simulink model "problem_7"  (R2020b)
settings: Solver=VariableStepAuto  StartTime=0.0  StopTime=10.0  RelTol=1e-3
values from neighbouring files (symbols this model uses):
  b11 = 1    [vars.m]
  b12 = 2    [vars.m]
  b13 = 1    [vars.m]
  b21 = 1    [vars.m]
  b22 = 1    [vars.m]
settings Model: Creator=hp  LastModifiedBy=hp

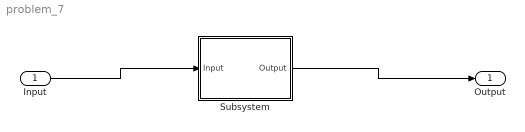
== system problem_7 ==
  Input : Inport
  Subsystem : Subsystem
  Output : Outport
  wires:
  Input/1 -> Subsystem/1(Input)
  Subsystem/1(Output) -> Output/1

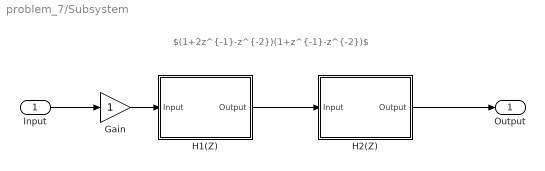
== system problem_7/Subsystem ==
  note: $(1+2z^{-1}-z^{-2})(1+z^{-1}-z^{-2})$
  Input : Inport
  Gain : Gain
  H1(Z) : Subsystem
  H2(Z) : Subsystem
  Output : Outport
  wires:
  H1(Z)/1(Output) -> H2(Z)/1(Input)
  H2(Z)/1(Output) -> Output/1
  Input/1 -> Gain/1
  Gain/1 -> H1(Z)/1(Input)

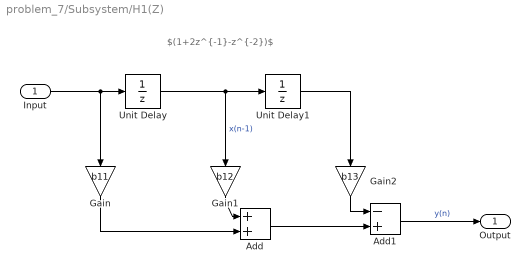
== system problem_7/Subsystem/H1(Z) ==
  note: $(1+2z^{-1}-z^{-2})$
  Input : Inport
  Add : Sum
  Add1 : Sum  Inputs=-+
  Gain : Gain  Gain=b11
  Gain1 : Gain  Gain=b12
  Gain2 : Gain  Gain=b13
  Unit Delay : UnitDelay  SampleTime=-1  HasFrameUpgradeWarning=on
  Unit Delay1 : UnitDelay  SampleTime=-1  HasFrameUpgradeWarning=on
  Output : Outport
  wires:
  Unit Delay1/1 -> Gain2/1
  Gain1/1 -> Add/1
  Add/1 -> Add1/2
  Gain/1 -> Add/2
  Unit Delay/1 -> Gain1/1, Unit Delay1/1  "x(n-1)"
  Input/1 -> Gain/1, Unit Delay/1
  Gain2/1 -> Add1/1
  Add1/1 -> Output/1  "y(n)"

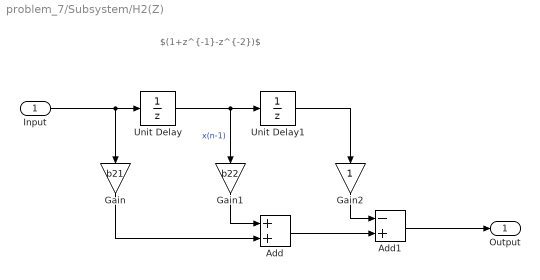
== system problem_7/Subsystem/H2(Z) ==
  note: $(1+z^{-1}-z^{-2})$
  Input : Inport
  Add : Sum
  Add1 : Sum  Inputs=-+
  Gain : Gain  Gain=b21
  Gain1 : Gain  Gain=b22
  Gain2 : Gain
  Unit Delay : UnitDelay  SampleTime=-1  HasFrameUpgradeWarning=on
  Unit Delay1 : UnitDelay  SampleTime=-1  HasFrameUpgradeWarning=on
  Output : Outport
  wires:
  Unit Delay/1 -> Gain1/1, Unit Delay1/1  "x(n-1)"
  Input/1 -> Gain/1, Unit Delay/1
  Add1/1 -> Output/1
  Gain/1 -> Add/2
  Unit Delay1/1 -> Gain2/1
  Add/1 -> Add1/2
  Gain2/1 -> Add1/1
  Gain1/1 -> Add/1
